simulink model "Q8_simulink"  (R2020b)
settings: Solver=VariableStepAuto  StartTime=0.0  StopTime=800  RelTol=1e-3
values from neighbouring files (symbols this model uses):
  Cz = minreal(Cz)    [Q7.m]    (also in Q8.m)
  Cz1 = simplifyFraction(Cz1)    [Q3.m]    (also in Q8.m = tf([-80351 80249],[10000 -10000],5))
  Cz2 = vpa(subs(Cz2,T,Ts))    [Q3.m]    (also in Q8.m = double(k)*tf([1 -exp(-(0.00204/8.03)*Ts)],[1 -1],5))
  Hs = tf(-4.875e-6,[1 0.1173 0.002308 0])    [Q8.m]
  Hz = c2d(H,5,'zoh')    [Q4.m]    (also in Q5.m; Q6.m; Q7.m; Q8.m = c2d(Hs,5,'zoh'))
libraries: simulink x1
settings Model: Creator=User  LastModifiedBy=User

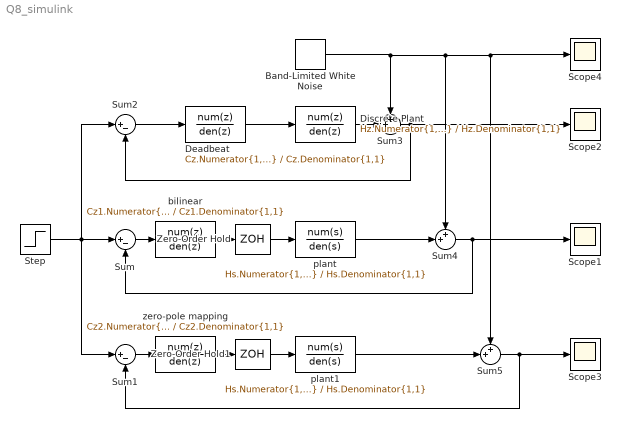
== system Q8_simulink ==
  Band-Limited White Noise : simulink/Sources/Band-Limited White Noise  Cov=[0.01]  Ts=5  seed=[23341]
  "Deadbeat " : DiscreteTransferFcn  Numerator=Cz.Numerator{1,1}  Denominator=Cz.Denominator{1,1}  SampleTime=5
  Discrete Plant : DiscreteTransferFcn  Numerator=Hz.Numerator{1,1}  Denominator=Hz.Denominator{1,1}
  Scope{1..4} (4 alike) : Scope
  Step : Step  SampleTime=0
  Sum : Sum  Inputs=|+-
  Sum1 : Sum  Inputs=|+-
  Sum2 : Sum  Inputs=|+-
  Sum3 : Sum  Inputs=++|
  Sum4 : Sum  Inputs=++|
  Sum5 : Sum  Inputs=++|
  Zero-Order Hold : ZeroOrderHold  SampleTime=5
  Zero-Order Hold1 : ZeroOrderHold  SampleTime=5
  bilinear : DiscreteTransferFcn  Numerator=Cz1.Numerator{1,1}  Denominator=Cz1.Denominator{1,1}  SampleTime=5
  plant : TransferFcn  Numerator=Hs.Numerator{1,1}  Denominator=Hs.Denominator{1,1}
  plant1 : TransferFcn  Numerator=Hs.Numerator{1,1}  Denominator=Hs.Denominator{1,1}
  zero-pole mapping : DiscreteTransferFcn  Numerator=Cz2.Numerator{1,1}  Denominator=Cz2.Denominator{1,1}  SampleTime=5
  wires:
  "Deadbeat "/1 -> Discrete Plant/1
  zero-pole mapping/1 -> Zero-Order Hold1/1
  bilinear/1 -> Zero-Order Hold/1
  Sum/1 -> bilinear/1
  Sum1/1 -> zero-pole mapping/1
  Step/1 -> Sum2/1, Sum1/1, Sum/1
  Sum2/1 -> "Deadbeat "/1
  Zero-Order Hold/1 -> plant/1
  Zero-Order Hold1/1 -> plant1/1
  Discrete Plant/1 -> Sum3/2
  Sum3/1 -> Scope2/1, Sum2/2
  Band-Limited White Noise/1 -> Sum4/1, Scope4/1, Sum5/1, Sum3/1
  plant/1 -> Sum4/2
  plant1/1 -> Sum5/2
  Sum5/1 -> Sum1/2, Scope3/1
  Sum4/1 -> Sum/2, Scope1/1
